simulink model "mmjd"  (R2014a)
settings: Solver=ode45  StartTime=0.0  StopTime=0.1  RelTol=1e-3
values from neighbouring files (symbols this model uses):
  C = 1e-6    (= 1e-06)    [sss.m]
  f = 1e3    (= 1000)    [sss.m]
  L = 5e-3    (= 0.005)    [sss.m]
  R1 = 4.7e3    (= 4700)    [sss.m]
  R2 = 3.6e3    (= 3600)    [sss.m]
  Vm = 10    [sss.m]
settings Model: Creator=Diana  LastModifiedBy=Diana

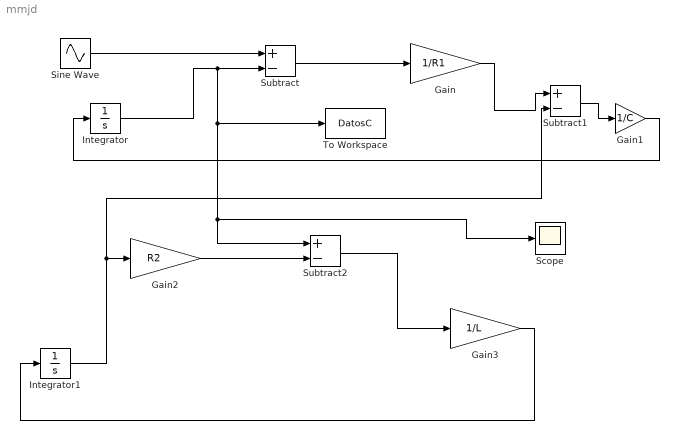
== system mmjd ==
  Gain : Gain  Gain=1/R1
  Gain1 : Gain  Gain=1/C
  Gain2 : Gain  Gain=R2
  Gain3 : Gain  Gain=1/L
  Integrator : Integrator
  Integrator1 : Integrator
  Scope : Scope
  Sine Wave : Sin  Amplitude=Vm  Frequency=2*pi*f  SampleTime=0
  Subtract : Sum  Inputs=+-
  Subtract1 : Sum  Inputs=+-
  Subtract2 : Sum  Inputs=+-
  To Workspace : ToWorkspace  VariableName=DatosC  SaveFormat=Timeseries  SampleTime=-1
  wires:
  Sine Wave/1 -> Subtract/1
  Subtract/1 -> Gain/1
  Gain/1 -> Subtract1/1
  Integrator1/1 -> Subtract1/2, Gain2/1
  Subtract1/1 -> Gain1/1
  Gain1/1 -> Integrator/1
  Integrator/1 -> To Workspace/1, Scope/1, Subtract2/1, Subtract/2
  Gain2/1 -> Subtract2/2
  Subtract2/1 -> Gain3/1
  Gain3/1 -> Integrator1/1
